simulink model "nlmodelLIN"  (R2020a)
settings: Solver=FixedStepAuto  StartTime=0.0  StopTime=5401  RelTol=1e-3
values from neighbouring files (symbols this model uses):
  alpha1hat = 0.0114    [Linearize_whitebox.m]    (also in Linearize_whitebox_final.m; lqr_whitebox.mat; matrices.mat)
  alpha2hat = 0.0079    [Linearize_whitebox.m]    (also in Linearize_whitebox_final.m; lqr_whitebox.mat; matrices.mat)
  areahat = 0.0009    [Linearize_whitebox.m]    (also in Linearize_whitebox_final.m; lqr_whitebox.mat; matrices.mat)
  areashat = 0.0004    [Linearize_whitebox.m]    (also in Linearize_whitebox_final.m; lqr_whitebox.mat; matrices.mat)
  boltz = 5.67e-8    (= 5.67e-08)    [Linearize_whitebox.m]    (also in Linearize_whitebox_final.m; lqr_whitebox.mat; matrices.mat; nonlinid.m)
  cphat = 501.9208    [Linearize_whitebox.m]    (also in Linearize_whitebox_final.m; lqr_whitebox.mat; matrices.mat)
  emishat = 0.9000    (= 0.9)    [Linearize_whitebox.m]    (also in Linearize_whitebox_final.m; lqr_whitebox.mat; matrices.mat)
  masshat = 0.0052    [Linearize_whitebox.m]    (also in Linearize_whitebox_final.m; lqr_whitebox.mat; matrices.mat)
  Tamb1 = 273.15+19.4037+7    (= 299.5537)    [Linearize_whitebox.m]    (also in Linearize_whitebox_final.m; lqr_whitebox.mat; matrices.mat; model.m = 26.4037)
  Tamb2 = 273.15+18.4262+6.5    (= 298.0762)    [Linearize_whitebox.m]    (also in Linearize_whitebox_final.m; lqr_whitebox.mat; matrices.mat; model.m = 24.9262)
  tauhat = 24.4408    [Linearize_whitebox.m]    (also in Linearize_whitebox_final.m; lqr_whitebox.mat; matrices.mat)
  uhat = 10.2021    [Linearize_whitebox.m]    (also in Linearize_whitebox_final.m; lqr_whitebox.mat; matrices.mat)
  ushat = 13.8985    [Linearize_whitebox.m]    (also in Linearize_whitebox_final.m; lqr_whitebox.mat; matrices.mat)
  x0 = [y1(1);y2(1)]    [Linearize_whitebox.m]    (also in Linearize_whitebox_final.m; lqr_whitebox.mat = [0 0]; matrices.mat = [293.042473118 292.064956012]; nonlinid.m)
settings Model: Creator=Eveline  LastModifiedBy=Eveline
settings DataIOCC: ExternalInput=U1, U2  ReturnWorkspaceOutputs=off  StateSaveName=xm  TimeSaveName=tm
settings DebuggingCC: AlgebraicLoopMsg=none  ArtificialAlgebraicLoopMsg=none  ModelReferenceExtraNoncontSigs=none  OperatingPointInterfaceChecksumMismatchMsg=none

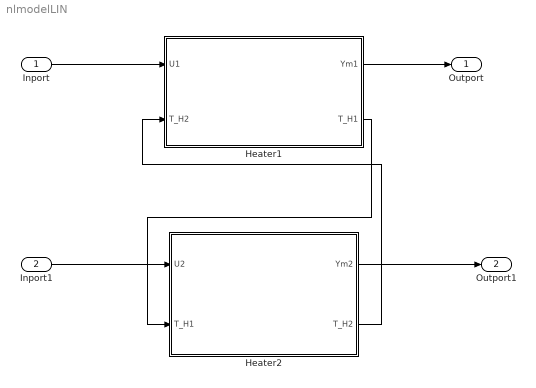
== system nlmodelLIN ==
  Inport : Inport
  Inport1 : Inport  Port=2
  Heater1 : Subsystem
  Heater2 : Subsystem
  Outport : Outport
  Outport1 : Outport  Port=2
  wires:
  Inport/1 -> Heater1/1(U1)
  Heater1/1(Ym1) -> Outport/1
  Inport1/1 -> Heater2/1(U2)
  Heater1/2(T_H1) -> Heater2/2(T_H1)
  Heater2/2(T_H2) -> Heater1/2(T_H2)
  Heater2/1(Ym2) -> Outport1/1

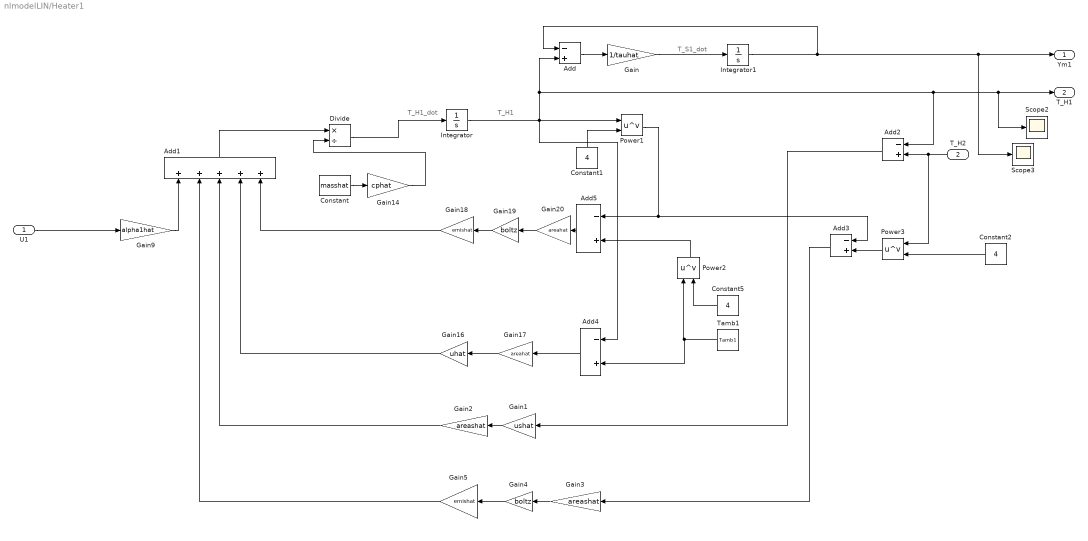
== system nlmodelLIN/Heater1 ==
  note: T_S1_dot
  note: T_H1
  note: T_H1_dot
  U1 : Inport
  T_H2 : Inport  Port=2
  Add{,2..5} (5 alike) : Sum  Inputs=-+
  Add1 : Sum  Inputs=+++++
  Constant : Constant  Value=masshat
  Constant1 : Constant  Value=4
  Constant2 : Constant  Value=4
  Constant5 : Constant  Value=4
  Divide : Product  Inputs=*/
  Gain : Gain  Gain=1/tauhat
  Gain1 : Gain  Gain=ushat
  Gain14 : Gain  Gain=cphat
  Gain16 : Gain  Gain=uhat
  Gain17 : Gain  Gain=areahat
  Gain18 : Gain  Gain=emishat
  Gain19 : Gain  Gain=boltz
  Gain2 : Gain  Gain=areashat
  Gain20 : Gain  Gain=areahat
  Gain3 : Gain  Gain=areashat
  Gain4 : Gain  Gain=boltz
  Gain5 : Gain  Gain=emishat
  Gain9 : Gain  Gain=alpha1hat
  Integrator : Integrator  InitialCondition=x0(1)
  Integrator1 : Integrator  InitialCondition=x0(1)
  Power1 : Math  Operator=pow  SaturateOnIntegerOverflow=on
  Power2 : Math  Operator=pow  SaturateOnIntegerOverflow=on
  Power3 : Math  Operator=pow  SaturateOnIntegerOverflow=on
  Scope2 : Scope
  Scope3 : Scope
  Tamb1 : Constant  Value=Tamb1  SampleTime=0
  Ym1 : Outport
  T_H1 : Outport  Port=2
  wires:
  Add/1 -> Gain/1
  Gain17/1 -> Gain16/1
  Constant5/1 -> Power2/2
  Integrator/1 -> Add4/1, Add2/1, Scope2/1, T_H1/1, Add/2, Power1/1
  Constant1/1 -> Power1/2
  Add5/1 -> Gain20/1
  Add1/1 -> Divide/1
  Add4/1 -> Gain17/1
  Gain20/1 -> Gain19/1
  Tamb1/1 -> Add4/2, Power2/1
  Divide/1 -> Integrator/1
  Power2/1 -> Add5/2
  Power1/1 -> Add3/1, Add5/1
  Gain19/1 -> Gain18/1
  Gain18/1 -> Add1/5
  Gain9/1 -> Add1/1
  Gain16/1 -> Add1/4
  Gain1/1 -> Gain2/1
  T_H2/1 -> Power3/1, Add2/2
  Add2/1 -> Gain1/1
  Gain2/1 -> Add1/3
  Constant2/1 -> Power3/2
  Power3/1 -> Add3/2
  Gain4/1 -> Gain5/1
  Gain3/1 -> Gain4/1
  Add3/1 -> Gain3/1
  Gain5/1 -> Add1/2
  U1/1 -> Gain9/1
  Constant/1 -> Gain14/1
  Gain14/1 -> Divide/2
  Gain/1 -> Integrator1/1
  Integrator1/1 -> Add/1, Scope3/1, Ym1/1

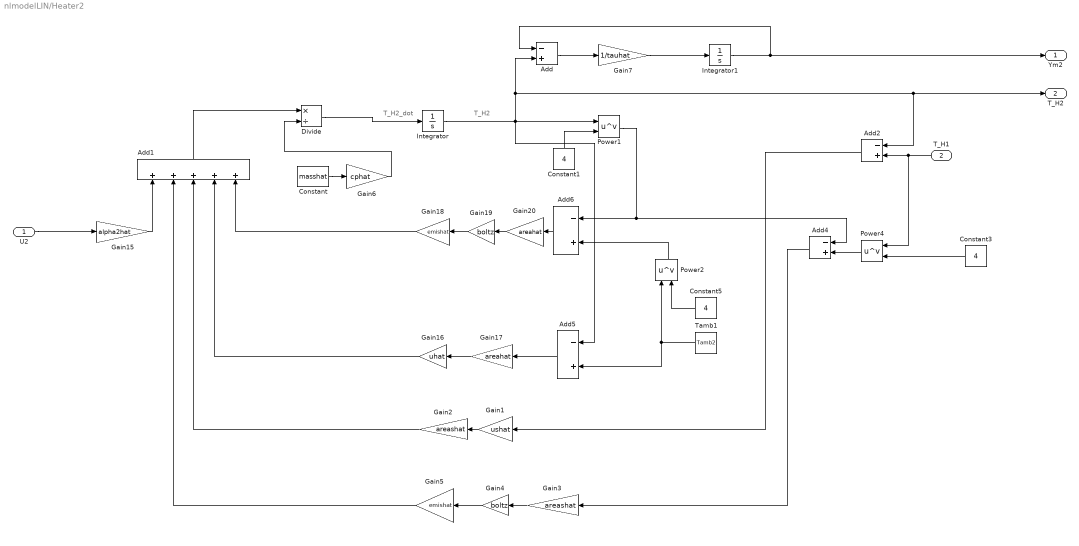
== system nlmodelLIN/Heater2 ==
  note: T_H2
  note: T_H2_dot
  U2 : Inport
  T_H1 : Inport  Port=2
  Add{,2,4..6} (5 alike) : Sum  Inputs=-+
  Add1 : Sum  Inputs=+++++
  Constant : Constant  Value=masshat
  Constant1 : Constant  Value=4
  Constant3 : Constant  Value=4
  Constant5 : Constant  Value=4
  Divide : Product  Inputs=*/
  Gain1 : Gain  Gain=ushat
  Gain15 : Gain  Gain=alpha2hat
  Gain16 : Gain  Gain=uhat
  Gain17 : Gain  Gain=areahat
  Gain18 : Gain  Gain=emishat
  Gain19 : Gain  Gain=boltz
  Gain2 : Gain  Gain=areashat
  Gain20 : Gain  Gain=areahat
  Gain3 : Gain  Gain=areashat
  Gain4 : Gain  Gain=boltz
  Gain5 : Gain  Gain=emishat
  Gain6 : Gain  Gain=cphat
  Gain7 : Gain  Gain=1/tauhat
  Integrator : Integrator  InitialCondition=x0(2)
  Integrator1 : Integrator  InitialCondition=x0(2)
  Power1 : Math  Operator=pow  SaturateOnIntegerOverflow=on
  Power2 : Math  Operator=pow  SaturateOnIntegerOverflow=on
  Power4 : Math  Operator=pow  SaturateOnIntegerOverflow=on
  Tamb1 : Constant  Value=Tamb2  SampleTime=0
  Ym2 : Outport
  T_H2 : Outport  Port=2
  wires:
  Gain17/1 -> Gain16/1
  Power4/1 -> Add4/2
  Gain20/1 -> Gain19/1
  Tamb1/1 -> Add5/2, Power2/1
  Constant3/1 -> Power4/2
  Integrator/1 -> Add5/1, T_H2/1, Add2/1, Add/2, Power1/1
  Add6/1 -> Gain20/1
  Gain1/1 -> Gain2/1
  Add4/1 -> Gain3/1
  Gain18/1 -> Add1/5
  Power2/1 -> Add6/2
  Add/1 -> Gain7/1
  Gain4/1 -> Gain5/1
  Constant1/1 -> Power1/2
  Add2/1 -> Gain1/1
  Constant5/1 -> Power2/2
  Add5/1 -> Gain17/1
  Gain2/1 -> Add1/3
  Gain5/1 -> Add1/2
  T_H1/1 -> Power4/1, Add2/2
  Divide/1 -> Integrator/1
  Gain19/1 -> Gain18/1
  Gain16/1 -> Add1/4
  Gain3/1 -> Gain4/1
  Gain15/1 -> Add1/1
  U2/1 -> Gain15/1
  Gain6/1 -> Divide/2
  Constant/1 -> Gain6/1
  Add1/1 -> Divide/1
  Gain7/1 -> Integrator1/1
  Integrator1/1 -> Add/1, Ym2/1
  Power1/1 -> Add4/1, Add6/1
